simulink model "Motor_piero"  (R2022b)
settings: Solver=VariableStepAuto  StartTime=0.0  StopTime=10.0  RelTol=1e-3
libraries: arduinolib x6, simulink x2
settings Model: Creator=marqu  LastModifiedBy=marqu

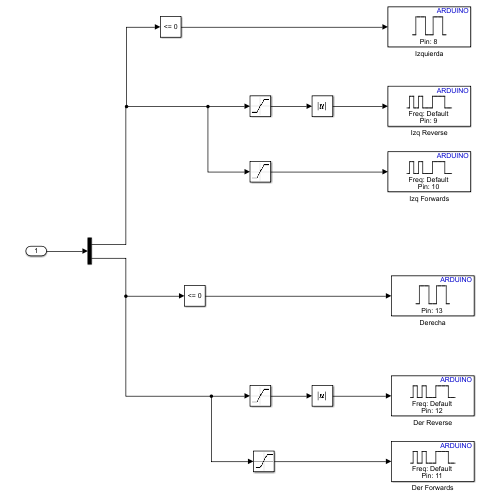
[thumbnail: Simulink's stored preview of the top-level diagram]
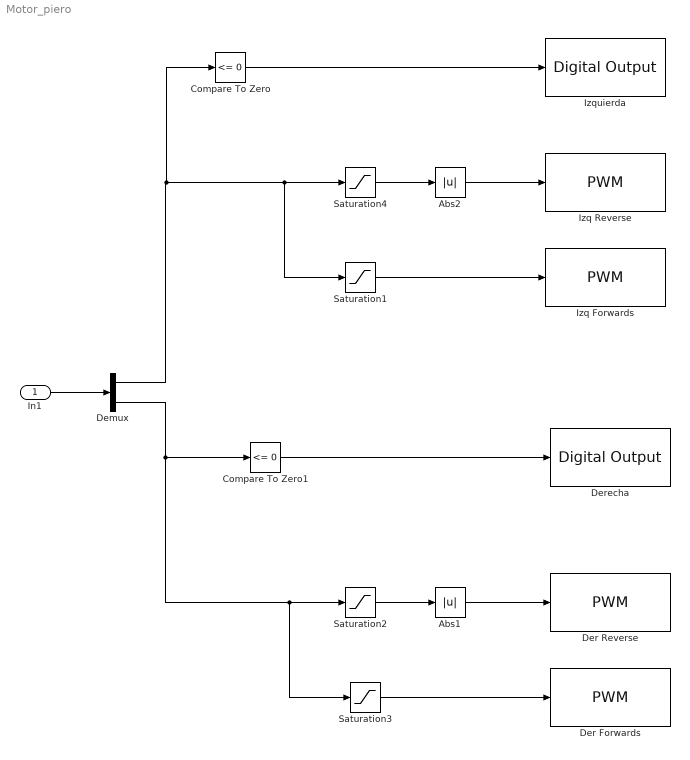
== system Motor_piero ==
  In1 : Inport
  Abs1 : Abs  SaturateOnIntegerOverflow=off
  Abs2 : Abs  SaturateOnIntegerOverflow=off
  Compare To Zero : simulink/Logic and Bit Operations/Compare To Zero  relop=<=  OutDataTypeStr=boolean
  Compare To Zero1 : simulink/Logic and Bit Operations/Compare To Zero  relop=<=  OutDataTypeStr=boolean
  Demux : Demux  Outputs=2
  Der Forwards : arduinolib/PWM  pinNumber=11  frequencyType=Default  desiredFrequency=490.2  achievableFrequency=490.2
  Der Reverse : arduinolib/PWM  pinNumber=12  frequencyType=Default  desiredFrequency=490.2  achievableFrequency=490.2
  Derecha : arduinolib/Digital Output  pinNumber=13  Direction=output  blockPlatform=arduino
  Izq Forwards : arduinolib/PWM  pinNumber=10  frequencyType=Default  desiredFrequency=490.2  achievableFrequency=490.2
  Izq Reverse : arduinolib/PWM  pinNumber=9  frequencyType=Default  desiredFrequency=490.2  achievableFrequency=490.2
  Izquierda : arduinolib/Digital Output  pinNumber=8  Direction=output  blockPlatform=arduino
  Saturation{1..4} (4 alike) : Saturate
  wires:
  Saturation4/1 -> Abs2/1
  Saturation2/1 -> Abs1/1
  Compare To Zero/1 -> Izquierda/1
  Demux/1 -> Compare To Zero/1, Saturation4/1, Saturation1/1
  In1/1 -> Demux/1
  Compare To Zero1/1 -> Derecha/1
  Abs2/1 -> Izq Reverse/1
  Abs1/1 -> Der Reverse/1
  Demux/2 -> Compare To Zero1/1, Saturation2/1, Saturation3/1
  Saturation3/1 -> Der Forwards/1
  Saturation1/1 -> Izq Forwards/1
